simulink model "Traffic"  (R2016b)
settings: Solver=FixedStepDiscrete  StartTime=0.0  StopTime=inf  RelTol=1e-3
model workspace (MAT data in the model file):
  Sig = Simulink.Signal
  Sig.DataType = 'boolean'
  Sig.Dimensions = -1
  Sig.DimensionsMode = 'auto'
  Sig.Complexity = 'auto'
  Sig.SampleTime = -1
  Sig.SamplingMode = 'auto'
  Sig1 = Simulink.Signal
  Sig1.DataType = 'boolean'
  Sig1.Dimensions = -1
  Sig1.DimensionsMode = 'auto'
  Sig1.Complexity = 'auto'
  Sig1.SampleTime = -1
  Sig1.SamplingMode = 'auto'
  Sig2 = Simulink.Signal
  Sig2.DataType = 'boolean'
  Sig2.Dimensions = -1
  Sig2.DimensionsMode = 'auto'
  Sig2.Complexity = 'auto'
  Sig2.SampleTime = -1
  Sig2.SamplingMode = 'auto'
  Sig3 = Simulink.Signal
  Sig3.DataType = 'auto'
  Sig3.Dimensions = -1
  Sig3.DimensionsMode = 'auto'
  Sig3.Complexity = 'auto'
  Sig3.SampleTime = -1
  Sig3.SamplingMode = 'auto'
settings Model: Creator=3essawy  LastModifiedBy=3essawy
settings OptimizationCC: DefaultParameterBehavior=Inlined
settings DebuggingCC: ParameterTunabilityLossMsg=error
settings RTWCC: SystemTargetFile=ert.tlc  GenCodeOnly=on  TemplateMakefile=ert_default_tmf  Description=Embedded Coder  GenerateReport=on  IncludeHyperlinkInReport=on  LaunchReport=on  GenerateTraceInfo=on  GenerateTraceReport=on  GenerateTraceReportSl=on  GenerateTraceReportSf=on  GenerateTraceReportEml=on
settings CodeAppCC: ForceParamTrailComments=on  IgnoreCustomStorageClasses=off  OperatorAnnotations=on  SimulinkDataObjDesc=on  SFDataObjDesc=on  MATLABFcnDesc=on  InsertBlockDesc=on  MATLABSourceComments=on
settings ERTTargetCC: TargetLangStandard=C99 (ISO)  GenerateSampleERTMain=on  InlinedParameterPlacement=NonHierarchical  ERTCustomFileTemplate=example_file_process.tlc  EnableUserReplacementTypes=on

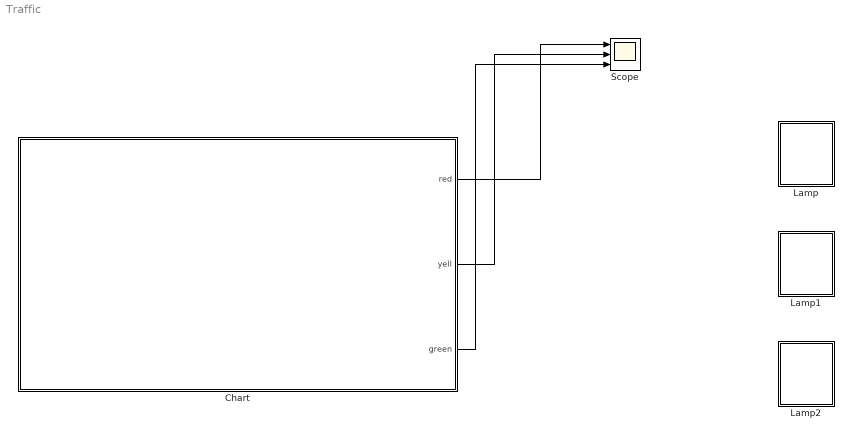
== system Traffic ==
  Chart : Stateflow chart  TreatAsAtomicUnit=on
  Lamp : Subsystem  DialogController=hmiCreateDDGDialog  IsWebBlock=on  mask(MWDashboardBlock){webBlockId=8ce7bbd7-da9e-4b0f-bcf8-31c68d10bd5c, webBlockType=lamp, ShowInLibBrowser=on, ShowInitialText=on, HMISrcModelName=Traffic}
      mask prompts: webBlockType "WebBlock Type"; HMISrcModelName "Source Model"
      mask help: SimulinkHMI:dialogs:LampDialogDesc
      mask Help: helpview([docroot '/mapfiles/simulink.map'], 'hmi_lamp')
      mask Display:
      | if strcmp(get_param(bdroot(gcb),'BlockDiagramType'), 'library')
      |     image([(matlabroot) '/toolbox/simulink/hmi/icons/Lamp.png']);
      | end
  Lamp1 : Subsystem  DialogController=hmiCreateDDGDialog  IsWebBlock=on  mask(MWDashboardBlock){webBlockId=17341ef9-bb8f-4ee7-8db5-d77e49a9e67c, webBlockType=lamp, ShowInLibBrowser=on, ShowInitialText=on, HMISrcModelName=Traffic}
      mask prompts: webBlockType "WebBlock Type"; HMISrcModelName "Source Model"
      mask help: SimulinkHMI:dialogs:LampDialogDesc
      mask Help: helpview([docroot '/mapfiles/simulink.map'], 'hmi_lamp')
      mask Display:
      | if strcmp(get_param(bdroot(gcb),'BlockDiagramType'), 'library')
      |     image([(matlabroot) '/toolbox/simulink/hmi/icons/Lamp.png']);
      | end
  Lamp2 : Subsystem  DialogController=hmiCreateDDGDialog  IsWebBlock=on  mask(MWDashboardBlock){webBlockId=dd92ffdc-1a79-4fad-8d13-8a4f13cd5c2c, webBlockType=lamp, ShowInLibBrowser=on, ShowInitialText=on, HMISrcModelName=Traffic}
      mask prompts: webBlockType "WebBlock Type"; HMISrcModelName "Source Model"
      mask help: SimulinkHMI:dialogs:LampDialogDesc
      mask Help: helpview([docroot '/mapfiles/simulink.map'], 'hmi_lamp')
      mask Display:
      | if strcmp(get_param(bdroot(gcb),'BlockDiagramType'), 'library')
      |     image([(matlabroot) '/toolbox/simulink/hmi/icons/Lamp.png']);
      | end
  Scope : Scope  NumInputPorts=3
  wires:
  Chart/1(red) -> Scope/1
  Chart/2(yell) -> Scope/2
  Chart/3(green) -> Scope/3

== system Traffic/Lamp ==

== system Traffic/Lamp1 ==

== system Traffic/Lamp2 ==

== stateflow chart Traffic/Chart ==
  state Stop
    entry:
    red=1;
    yell=0;
    green=0;
  state Prep
    entry:
    red=0;
    yell=1;
    green=0;
  state Go
    entry:
    red=0;
    yell=0;
    green=1;
  (default) -> Stop : {red=0;
      | yell=0;
      | green=0;}
  Stop -> Prep : after(20,sec)
  Prep -> Go : after(20,sec)
  Go -> Stop : after(20,sec)
  data: red output; yell output; green output
